simulink model "attitude_control"  (R2022b)
settings: Solver=VariableStepAuto  StartTime=0.0  StopTime=10.0  RelTol=1e-3
undefined symbols (not defined in the file): MAV
libraries: checkpacklib x2, slpidlib x2
settings Model: Creator=Tamer  LastModifiedBy=Tamer
settings SolverCC: ZeroCrossControl=DisableAll  AlgebraicLoopSolver=TrustRegion
settings DataIOCC: SaveOutput=off  SaveTime=off
settings DebuggingCC: UnconnectedInputMsg=warning  UnconnectedOutputMsg=warning  UnconnectedLineMsg=warning  SFMachineParentedDataDiag=warning
settings ModelReferenceCC: EnableRefExpFcnMdlSchedulingChecks=on
settings GRTTargetCC: CombineOutputUpdateFcns=off  MatFileLogging=off

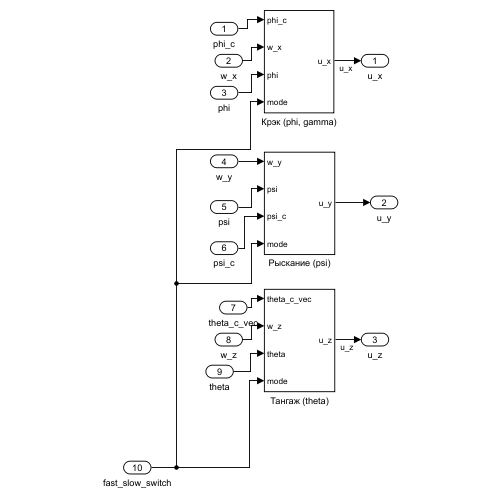
[thumbnail: Simulink's stored preview of the top-level diagram]
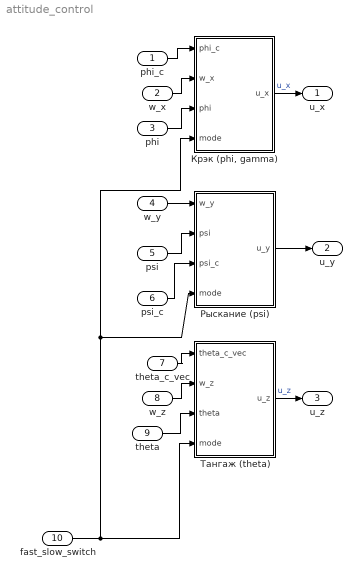
== system attitude_control ==
  phi_c : Inport
  w_x : Inport  Port=2
  phi : Inport  Port=3
  w_y : Inport  Port=4
  psi : Inport  Port=5
  psi_c : Inport  Port=6
  theta_c_vec : Inport  Port=7
  w_z : Inport  Port=8
  theta : Inport  Port=9
  fast_slow_switch : Inport  Port=10
  "Крэк (phi, gamma)" : Subsystem
      settings: PortSchema="{\"entries\":[{\"content\":{\"sides\":[{\"content\":{\"connectorIds\":[]},\"type\":\"ConnectorPlacement.EquallySpacedRectSide\",\"uuid\":\"a258f665-a86a-4482-bd07-3187ea478656\"},{\"content\":{\"connectorIds\":[],\"side\":\"RIGHT\"},\"type\":\"ConnectorPlacement.EquallySpacedRectSide\",\"uuid\":\"4cc1ffc1-e5d7-4190-ba75-89ce977e4acc\"},{\"content\":{\"connectorIds\":[\"Out1\"],\"side\":\"TOP\"},\"type\":\"ConnectorPlacement.EquallySpacedRectSide\",\"uuid\":\"daf9489c-9fb9-498c-b344-dda7a980194c\"},{\"content\":{\"connectorIds\":[\"In1\",\"In2\",\"In3\",\"In4\"],\"side\":\"BOTTOM\"},\"type\":\"ConnectorPlacement.EquallySpacedRectSide\",\"uuid\":\"f778d476-c858-4cc3-a786-5ff47391ec3b\"}]},\"type\":\"ConnectorPlacement.EquallySpacedConnector\",\"uuid\":\"5a79eedc-deb4-47bd-85cd-0d2cb0ea5802\"}],\"packageUris\":[\"http://schema.mathworks.com/mf0/Connector/R2020b\"],\"version\":\"1.0\"}"
  Рыскание (psi) : Subsystem
      settings: PortSchema="{\"entries\":[{\"content\":{\"sides\":[{\"content\":{\"connectorIds\":[]},\"type\":\"ConnectorPlacement.EquallySpacedRectSide\",\"uuid\":\"a258f665-a86a-4482-bd07-3187ea478656\"},{\"content\":{\"connectorIds\":[],\"side\":\"RIGHT\"},\"type\":\"ConnectorPlacement.EquallySpacedRectSide\",\"uuid\":\"4cc1ffc1-e5d7-4190-ba75-89ce977e4acc\"},{\"content\":{\"connectorIds\":[\"Out1\"],\"side\":\"TOP\"},\"type\":\"ConnectorPlacement.EquallySpacedRectSide\",\"uuid\":\"daf9489c-9fb9-498c-b344-dda7a980194c\"},{\"content\":{\"connectorIds\":[\"In1\",\"In2\",\"In3\",\"In4\"],\"side\":\"BOTTOM\"},\"type\":\"ConnectorPlacement.EquallySpacedRectSide\",\"uuid\":\"f778d476-c858-4cc3-a786-5ff47391ec3b\"}]},\"type\":\"ConnectorPlacement.EquallySpacedConnector\",\"uuid\":\"5a79eedc-deb4-47bd-85cd-0d2cb0ea5802\"}],\"packageUris\":[\"http://schema.mathworks.com/mf0/Connector/R2020b\"],\"version\":\"1.0\"}"
  Тангаж (theta) : Subsystem
      settings: PortSchema="{\"entries\":[{\"content\":{\"sides\":[{\"content\":{\"connectorIds\":[]},\"type\":\"ConnectorPlacement.EquallySpacedRectSide\",\"uuid\":\"a258f665-a86a-4482-bd07-3187ea478656\"},{\"content\":{\"connectorIds\":[],\"side\":\"RIGHT\"},\"type\":\"ConnectorPlacement.EquallySpacedRectSide\",\"uuid\":\"4cc1ffc1-e5d7-4190-ba75-89ce977e4acc\"},{\"content\":{\"connectorIds\":[\"Out1\"],\"side\":\"TOP\"},\"type\":\"ConnectorPlacement.EquallySpacedRectSide\",\"uuid\":\"daf9489c-9fb9-498c-b344-dda7a980194c\"},{\"content\":{\"connectorIds\":[\"In1\",\"In2\",\"In3\",\"In4\"],\"side\":\"BOTTOM\"},\"type\":\"ConnectorPlacement.EquallySpacedRectSide\",\"uuid\":\"f778d476-c858-4cc3-a786-5ff47391ec3b\"}]},\"type\":\"ConnectorPlacement.EquallySpacedConnector\",\"uuid\":\"5a79eedc-deb4-47bd-85cd-0d2cb0ea5802\"}],\"packageUris\":[\"http://schema.mathworks.com/mf0/Connector/R2020b\"],\"version\":\"1.0\"}"
  u_x : Outport
  u_y : Outport  Port=2
  u_z : Outport  Port=3
  wires:
  phi_c/1 -> "Крэк (phi, gamma)"/1(phi_c)
  w_x/1 -> "Крэк (phi, gamma)"/2(w_x)
  phi/1 -> "Крэк (phi, gamma)"/3(phi)
  w_y/1 -> Рыскание (psi)/1(w_y)
  psi/1 -> Рыскание (psi)/2(psi)
  psi_c/1 -> Рыскание (psi)/3(psi_c)
  theta_c_vec/1 -> Тангаж (theta)/1(theta_c_vec)
  w_z/1 -> Тангаж (theta)/2(w_z)
  theta/1 -> Тангаж (theta)/3(theta)
  "Крэк (phi, gamma)"/1(u_x) -> u_x/1  "u_x"
  Рыскание (psi)/1(u_y) -> u_y/1
  Тангаж (theta)/1(u_z) -> u_z/1  "u_z"
  fast_slow_switch/1 -> Рыскание (psi)/4(mode), "Крэк (phi, gamma)"/4(mode), Тангаж (theta)/4(mode)

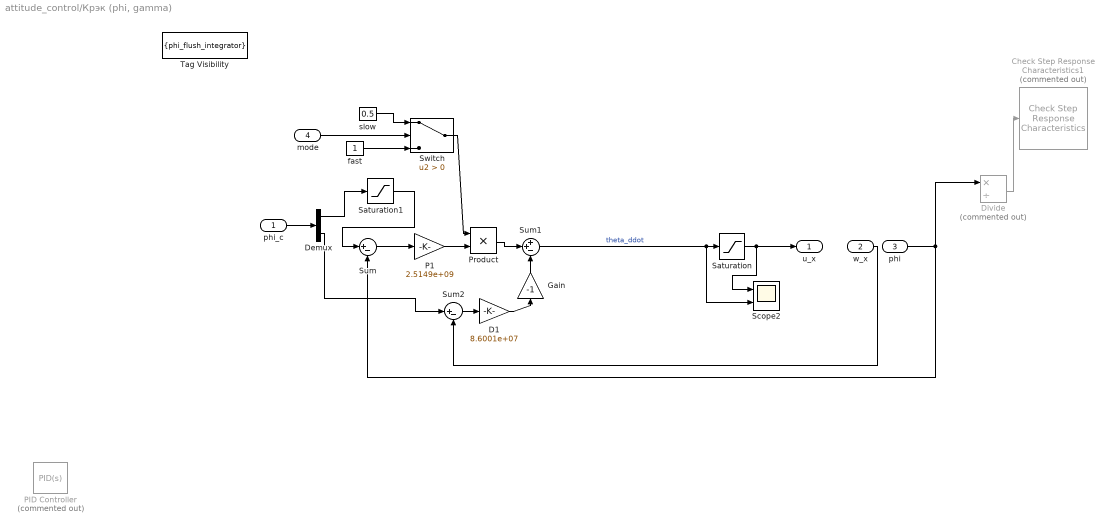
== system attitude_control/Крэк (phi, gamma) ==
  phi_c : Inport
  w_x : Inport  Port=2
  phi : Inport  Port=3
  mode : Inport  Port=4
  Check Step Response Characteristics1 : checkpacklib/Check Step Response  Characteristics  Commented=on  InstantiateOnLoad=on  enabled=off  stopWhenAssertionFail=off  export=off  ViewDlgPos=[358 -116 1306 720]  OpenViewOnLoad=off  LaunchViewOnOpen=off  TimeUnits=seconds  EnableStepResponseBound=on  InitialValue=0  FinalValue=1  StepTime=1  RiseTime=0.2  PercentRise=80  SettlingTime=0.5  PercentSettling=1  PercentOvershoot=10  PercentUndershoot=1
  D1 : Gain  Gain=8.6001e+07
  Demux : Demux  Outputs=2
  Divide : Product  Commented=on  Inputs=*/
  Gain : Gain  Gain=-1
  P1 : Gain  Gain=2.5149e+09
  PID Controller : slpidlib/PID Controller  Commented=on  Controller=PID  Form=Parallel  TimeDomain=Continuous-time  UseExternalTs=off  SampleTime=-1  IntegratorMethod=Forward Euler  FilterMethod=Forward Euler  ControllerParametersSource=internal  P=1  I=1  UseKiTs=off  D=0  N=100  UseFilter=on  TunerSelectOption=Transfer Function Based (PID Tuner App)  InitialConditionSource=internal  InitialConditionForIntegrator=0  InitialConditionForFilter=0  DifferentiatorICPrevScaledInput=0  ExternalReset=none  TrackingMode=off  Kt=1  LimitOutput=off  SatLimitsSource=internal  UpperSaturationLimit=inf  LowerSaturationLimit=-inf  LinearizeAsGain=on  AntiWindupMode=none  Kb=1  LimitIntegrator=off  UpperIntegratorSaturationLimit=inf  LowerIntegratorSaturationLimit=-inf  POutMin=[]  POutMax=[]  IOutMin=[]  IOutMax=[]  DOutMin=[]  DOutMax=[]  NOutMin=[]  NOutMax=[]  SumOutMin=[]  SumOutMax=[]  SaturationOutMin=[]  SaturationOutMax=[]  PParamMin=[]  PParamMax=[]  IParamMin=[]  IParamMax=[]  DParamMin=[]  DParamMax=[]  NParamMin=[]  NParamMax=[]  KbParamMin=[]  KbParamMax=[]  KtParamMin=[]  KtParamMax=[]  KbOutMin=[]  KbOutMax=[]  KtOutMin=[]  KtOutMax=[]  IntegratorOutMin=[]  IntegratorOutMax=[]  FilterOutMin=[]  FilterOutMax=[]  SumI1OutMin=[]  SumI1OutMax=[]  SumI2OutMin=[]  SumI2OutMax=[]  SumI3OutMin=[]  SumI3OutMax=[]  SumI4OutMin=[]  SumI4OutMax=[]  SumDOutMin=[]  SumDOutMax=[]  DifferentiatorOutMin=[]  DifferentiatorOutMax=[]  FilterDiffOutCoefMin=[]  FilterDiffOutCoefMax=[]  ReciprocalOutMin=[]  ReciprocalOutMax=[]  SumDenOutMin=[]  SumDenOutMax=[]  SumNumOutMin=[]  SumNumOutMax=[]  DivideOutMin=[]  DivideOutMax=[]  UdiffTsProdOutMin=[]  UdiffTsProdOutMax=[]  NTsProdOutMin=[]  NTsProdOutMax=[]  UintegralTsProdOutMin=[]  UintegralTsProdOutMax=[]  UngainTsProdOutMin=[]  UngainTsProdOutMax=[]  ClampingZeroOutDataTypeStr=Inherit: Inherit via back propagation  ClampingZeroOutMin=[]  ClampingZeroOutMax=[]  FilterDenConstantOutDataTypeStr=Inherit: Inherit via back propagation  FilterDenConstantOutMin=[]  FilterDenConstantOutMax=[]  PCopyOutDataTypeStr=Inherit: Inherit via back propagation  PCopyOutMin=[]  PCopyOutMax=[]  NCopyOutDataTypeStr=Inherit: Inherit via back propagation  NCopyOutMin=[]  NCopyOutMax=[]  IntegratorContinuousStateAttributes=''  IntegratorStateMustResolveToSignalObject=off  IntegratorRTWStateStorageClass=Auto  FilterContinuousStateAttributes=''  FilterStateMustResolveToSignalObject=off  FilterRTWStateStorageClass=Auto  ParallelPVariant=InternalParameters  IdealPVariant=Disabled  IVariant=InternalParameters  DVariant=InternalParameters  IntegratorVariant=Continuous  SatVariant=Disabled  AWVariant=Passthrough  PCopyVariant=Disabled  TRVariant=Disabled  FdbkBlocksVariant=Forward  IdealPFdbkVariant=Disabled  SatFdbkVariant=Disabled  DerivativeFilterVariant=ContFilter  NVariant=InternalParameters  NCopyVariant=Disabled  FilterICVariant=InternalICsFilter  IntegratorICVariant=InternalICs  ExternalResetVariant=Disabled  TRSumVariant=Passthrough  SumFdbkVariant=Disabled  SumVariant=Sum_PID  TsampFilterVariant=InternalTs  TsampNgainVariant=Passthrough  TsampIntegralVariant=Passthrough  ExternalSaturationOutDataTypeStr=Inherit: Same as second input
  Product : Product
  Saturation : Saturate  UpperLimit=MAV.Control.u_xz_max  LowerLimit=-MAV.Control.u_xz_max
  Saturation1 : Saturate  UpperLimit=deg2rad(90)  LowerLimit=-deg2rad(90)
  Scope2 : Scope  NumInputPorts=2
  Sum : Sum  Inputs=|+-
  Sum1 : Sum  Inputs=++-
  Sum2 : Sum  Inputs=|+-
  Switch : Switch  Criteria=u2 > Threshold  SaturateOnIntegerOverflow=off  InputSameDT=off
  Tag Visibility : GotoTagVisibility  GotoTag=phi_flush_integrator
  fast : Constant
  slow : Constant  Value=0.5
  u_x : Outport
  wires:
  Sum1/1 -> Saturation/1, Scope2/2  "theta_ddot"
  phi/1 -> Sum/2, Divide/1
  Saturation/1 -> Scope2/1, u_x/1
  Sum2/1 -> D1/1
  D1/1 -> Gain/1
  w_x/1 -> Sum2/2
  Gain/1 -> Sum1/3
  Divide/1 -> Check Step Response Characteristics1/1
  Sum/1 -> P1/1
  Demux/2 -> Sum2/1
  phi_c/1 -> Demux/1
  Demux/1 -> Saturation1/1
  Saturation1/1 -> Sum/1
  P1/1 -> Product/2
  Switch/1 -> Product/1
  mode/1 -> Switch/2
  fast/1 -> Switch/3
  slow/1 -> Switch/1
  Product/1 -> Sum1/2

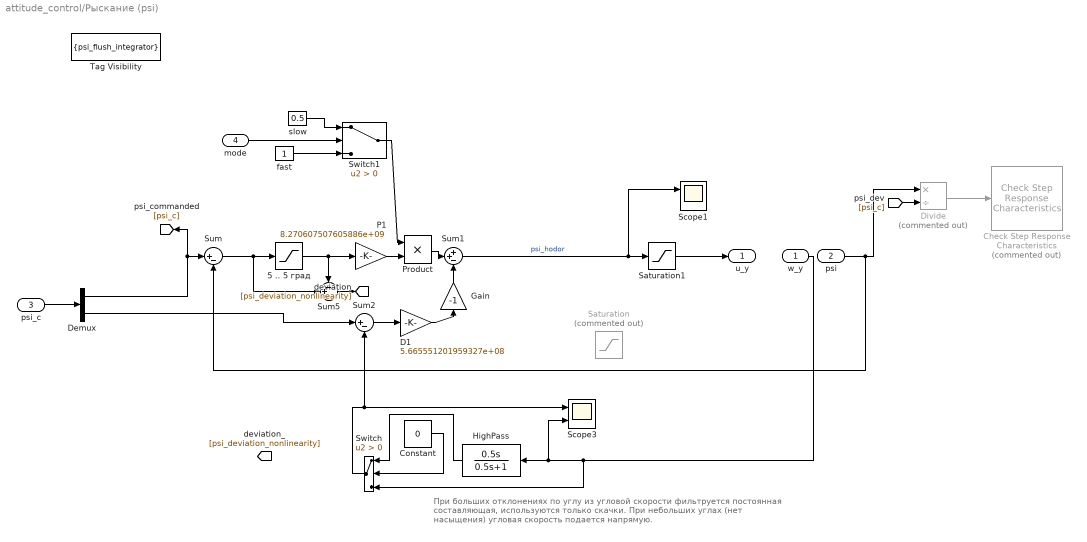
== system attitude_control/Рыскание (psi) ==
  note: При больших отклонениях по углу из угловой скорости фильтруется
      | постоянная составляющая, используются только скачки.
      | При небольших углах (нет насыщения) угловая скорость подается напрямую.
  w_y : Inport
  psi : Inport  Port=2
  psi_c : Inport  Port=3
  mode : Inport  Port=4
  5 .. 5 град : Saturate  UpperLimit=deg2rad(5)  LowerLimit=-deg2rad(5)
  Check Step Response Characteristics : checkpacklib/Check Step Response  Characteristics  Commented=on  InstantiateOnLoad=on  enabled=on  stopWhenAssertionFail=off  export=off  ViewDlgPos=[100 11 1618 919]  OpenViewOnLoad=off  LaunchViewOnOpen=off  TimeUnits=seconds  EnableStepResponseBound=on  InitialValue=0  FinalValue=1  StepTime=1  RiseTime=0.8  PercentRise=80  SettlingTime=1  PercentSettling=1  PercentOvershoot=4  PercentUndershoot=1
  Constant : Constant  Value=0
  D1 : Gain  Gain=5.665551201959327e+08
  Demux : Demux  Outputs=2
  Divide : Product  Commented=on  Inputs=*/
  Gain : Gain  Gain=-1
  HighPass : TransferFcn  Numerator=[0.5 0]  Denominator=[0.5 1]
  P1 : Gain  Gain=8.270607507605886e+09
  Product : Product
  Saturation : Saturate  Commented=on  UpperLimit=449800000  LowerLimit=-449800000
  Saturation1 : Saturate  UpperLimit=449800000  LowerLimit=-449800000
  Scope1 : Scope  NumInputPorts=2
  Scope3 : Scope  NumInputPorts=2
  Sum : Sum  Inputs=|+-
  Sum1 : Sum  Inputs=++-
  Sum2 : Sum  Inputs=|+-
  Sum5 : Sum  Inputs=-+|
  Switch : Switch  Criteria=u2 > Threshold  SaturateOnIntegerOverflow=off  InputSameDT=off
  Switch1 : Switch  Criteria=u2 > Threshold  SaturateOnIntegerOverflow=off  InputSameDT=off
  Tag Visibility : GotoTagVisibility  GotoTag=psi_flush_integrator
  fast : Constant
  slow : Constant  Value=0.5
  u_y : Outport
  wires:
  Sum1/1 -> Saturation1/1, Scope1/1  "psi_hodor"
  psi/1 -> Divide/1, Sum/2
  Saturation1/1 -> u_y/1
  Sum2/1 -> D1/1
  D1/1 -> Gain/1
  Divide/1 -> Check Step Response Characteristics/1
  Demux/1 -> [psi_c], Sum/1
  Demux/2 -> Sum2/1
  Sum/1 -> Sum5/2, 5 .. 5 град/1
  5 .. 5 град/1 -> P1/1, Sum5/1
  w_y/1 -> Switch/3, Scope3/2, HighPass/1
  Switch/1 -> Scope3/1, Sum2/2
  Sum5/1 -> [psi_deviation_nonlinearity]
  [psi_c] -> Divide/2
  Gain/1 -> Sum1/3
  Constant/1 -> Switch/2
  HighPass/1 -> Switch/1
  psi_c/1 -> Demux/1
  Switch1/1 -> Product/1
  fast/1 -> Switch1/3
  mode/1 -> Switch1/2
  slow/1 -> Switch1/1
  P1/1 -> Product/2
  Product/1 -> Sum1/2

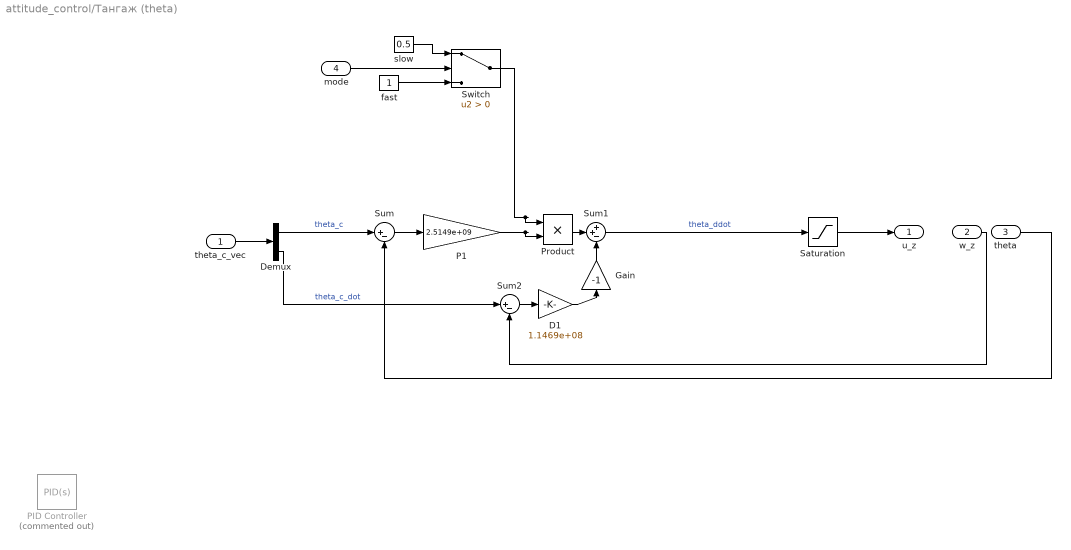
== system attitude_control/Тангаж (theta) ==
  theta_c_vec : Inport
  w_z : Inport  Port=2
  theta : Inport  Port=3
  mode : Inport  Port=4
  D1 : Gain  Gain=1.1469e+08
  Demux : Demux  Outputs=2
  Gain : Gain  Gain=-1
  P1 : Gain  Gain=2.5149e+09
  PID Controller : slpidlib/PID Controller  Commented=on  Controller=PID  Form=Parallel  TimeDomain=Continuous-time  UseExternalTs=off  SampleTime=-1  IntegratorMethod=Forward Euler  FilterMethod=Forward Euler  ControllerParametersSource=internal  P=1  I=1  UseKiTs=off  D=0  N=100  UseFilter=on  TunerSelectOption=Transfer Function Based (PID Tuner App)  InitialConditionSource=internal  InitialConditionForIntegrator=0  InitialConditionForFilter=0  DifferentiatorICPrevScaledInput=0  ExternalReset=none  TrackingMode=off  Kt=1  LimitOutput=off  SatLimitsSource=internal  UpperSaturationLimit=inf  LowerSaturationLimit=-inf  LinearizeAsGain=on  AntiWindupMode=none  Kb=1  LimitIntegrator=off  UpperIntegratorSaturationLimit=inf  LowerIntegratorSaturationLimit=-inf  POutMin=[]  POutMax=[]  IOutMin=[]  IOutMax=[]  DOutMin=[]  DOutMax=[]  NOutMin=[]  NOutMax=[]  SumOutMin=[]  SumOutMax=[]  SaturationOutMin=[]  SaturationOutMax=[]  PParamMin=[]  PParamMax=[]  IParamMin=[]  IParamMax=[]  DParamMin=[]  DParamMax=[]  NParamMin=[]  NParamMax=[]  KbParamMin=[]  KbParamMax=[]  KtParamMin=[]  KtParamMax=[]  KbOutMin=[]  KbOutMax=[]  KtOutMin=[]  KtOutMax=[]  IntegratorOutMin=[]  IntegratorOutMax=[]  FilterOutMin=[]  FilterOutMax=[]  SumI1OutMin=[]  SumI1OutMax=[]  SumI2OutMin=[]  SumI2OutMax=[]  SumI3OutMin=[]  SumI3OutMax=[]  SumI4OutMin=[]  SumI4OutMax=[]  SumDOutMin=[]  SumDOutMax=[]  DifferentiatorOutMin=[]  DifferentiatorOutMax=[]  FilterDiffOutCoefMin=[]  FilterDiffOutCoefMax=[]  ReciprocalOutMin=[]  ReciprocalOutMax=[]  SumDenOutMin=[]  SumDenOutMax=[]  SumNumOutMin=[]  SumNumOutMax=[]  DivideOutMin=[]  DivideOutMax=[]  UdiffTsProdOutMin=[]  UdiffTsProdOutMax=[]  NTsProdOutMin=[]  NTsProdOutMax=[]  UintegralTsProdOutMin=[]  UintegralTsProdOutMax=[]  UngainTsProdOutMin=[]  UngainTsProdOutMax=[]  ClampingZeroOutDataTypeStr=Inherit: Inherit via back propagation  ClampingZeroOutMin=[]  ClampingZeroOutMax=[]  FilterDenConstantOutDataTypeStr=Inherit: Inherit via back propagation  FilterDenConstantOutMin=[]  FilterDenConstantOutMax=[]  PCopyOutDataTypeStr=Inherit: Inherit via back propagation  PCopyOutMin=[]  PCopyOutMax=[]  NCopyOutDataTypeStr=Inherit: Inherit via back propagation  NCopyOutMin=[]  NCopyOutMax=[]  IntegratorContinuousStateAttributes=''  IntegratorStateMustResolveToSignalObject=off  IntegratorRTWStateStorageClass=Auto  FilterContinuousStateAttributes=''  FilterStateMustResolveToSignalObject=off  FilterRTWStateStorageClass=Auto  ParallelPVariant=InternalParameters  IdealPVariant=Disabled  IVariant=InternalParameters  DVariant=InternalParameters  IntegratorVariant=Continuous  SatVariant=Disabled  AWVariant=Passthrough  PCopyVariant=Disabled  TRVariant=Disabled  FdbkBlocksVariant=Forward  IdealPFdbkVariant=Disabled  SatFdbkVariant=Disabled  DerivativeFilterVariant=ContFilter  NVariant=InternalParameters  NCopyVariant=Disabled  FilterICVariant=InternalICsFilter  IntegratorICVariant=InternalICs  ExternalResetVariant=Disabled  TRSumVariant=Passthrough  SumFdbkVariant=Disabled  SumVariant=Sum_PID  TsampFilterVariant=InternalTs  TsampNgainVariant=Passthrough  TsampIntegralVariant=Passthrough  ExternalSaturationOutDataTypeStr=Inherit: Same as second input
  Product : Product
  Saturation : Saturate  UpperLimit=MAV.Control.u_xz_max  LowerLimit=-MAV.Control.u_xz_max
  Sum : Sum  Inputs=|+-
  Sum1 : Sum  Inputs=++-
  Sum2 : Sum  Inputs=|+-
  Switch : Switch  Criteria=u2 > Threshold  SaturateOnIntegerOverflow=off  InputSameDT=off
  fast : Constant
  slow : Constant  Value=0.5
  u_z : Outport
  wires:
  Sum/1 -> P1/1
  Sum1/1 -> Saturation/1  "theta_ddot"
  theta/1 -> Sum/2
  Saturation/1 -> u_z/1
  Sum2/1 -> D1/1
  D1/1 -> Gain/1
  w_z/1 -> Sum2/2
  Demux/2 -> Sum2/1  "theta_c_dot"
  Demux/1 -> Sum/1  "theta_c"
  theta_c_vec/1 -> Demux/1
  Gain/1 -> Sum1/3
  Switch/1 -> Product/1
  fast/1 -> Switch/3
  mode/1 -> Switch/2
  slow/1 -> Switch/1
  P1/1 -> Product/2
  Product/1 -> Sum1/2
